simulink model "ADU_Integration_Y2016_simulation"  (R2016b)
settings: Solver=FixedStepDiscrete  StartTime=240  StopTime=300  FixedStep=0.01  RelTol=1e-3  EnableMultiTasking=on
PostLoadFcn:
  | , if any(exist('dsrtsu_mdlpostloadfcn', 'file') == [2, 3, 6]), try dsrtsu_mdlpostloadfcn('Execute', bdroot); catch fprintf('Error in PostLoadFcn (dsrtsu_mdlpostloadfcn) for model "%s":\n %s\n', bdroot, lasterr); end, end,
InitFcn:
  | load 'data/chi2_dat';
  | load 'data/innerLine_struct';
  | load 'data/middleLine_struct';
  | load 'data/outerLine_struct';
  | load 'data/innerLine';
  | load 'data/middleLine';
  | load 'data/outerLine';
  | load 'data/landmarks_patac_schimmel_ccw';
  | load 'data/patac_navi_array';
  | load 'data/sensor';
  | load 'data/map_struct';
  | addpath map_src
  | Integration_Parameter;
  | load 'TestData_001';
values from neighbouring files (symbols this model uses):
  TestData_001 =     [TestData_001.mat]
undefined symbols (not defined in the file or in its folder): a, chi2_dat, innerLine, landmarks_patac_schimmel_ccw, middleLine, outerLine, patac_navi_array, StartNum
libraries: simulink x36, rtican x1
(part 18 of 20)

== stateflow chart ADU_Integration_Y2016_simulation/LogData/RR_SRR_Data/Chart ==
  (default) -> (junction 13)
  (junction 13) -> (junction 14) [order 1] : [Trig != preTrig]
  (junction 13) -> (junction 15) [order 2]
  (junction 14) -> (junction 16) : {
      | DataOutput=DataInput;
      | Time_out=Time;
      | }
  (junction 16) -> (junction 15)
  (junction 15) -> (junction 17) : {
      | preTrig=Trig;
      | }
  data: Trig input; DataInput input size=[10 5]; DataOutput output double size=[10 5]; Time input; preTrig local double; Time_out output double

== matlab function ADU_Integration_Y2016_simulation/Path_Plan1/InterSectionPathPlanningModule/PathPrePointCal/PrePointCal ==
  data: V_tar input; Delta input; Arclength input; T_long input; T_lat input; Info_Me input; x_in input; y_in input; angle_in input; x_out input; y_out input; angle_out input; Time input; quadsinu2tbl data_store_memory; quadcosu2tbl data_store_memory; xposition output; yposition output; Ax output; Ay output; Vx output; Vy output; Theta output; PathPlanRes input; PathTrjFinishFlg output
function [xposition,yposition,Ax,Ay,Vx,Vy,Theta,PathTrjFinishFlg] = ElementaryPosCal( V_tar,Delta,Arclength,T_long,T_lat,Info_Me,x_in,y_in,angle_in,x_out,y_out,angle_out,Time,PathPlanRes)
%UNTITLED Summary of this function goes here
%   Detailed explanation goes here
persistent PrePointCalEn
if isempty(PrePointCalEn)
    PrePointCalEn = 0;
end
if PrePointCalEn <1e-1
    if PathPlanRes > 1e-1
        PrePointCalEn = 1;
    end
end
xposition = 0;yposition = 0;Ax = 0;Ay = 0;Vx = 0;Vy = 0;Theta = 0;PathTrjFinishFlg = 0;
    if PrePointCalEn > 1e-1
        V_me = Info_Me(3);
        Arc = 255;
        V_tarPos = 255;
        if Time > T_lat
        else
            if Time <= T_long
                if abs(V_tar - V_me) >1e-5
                    a_me = (V_tar - V_me)/T_long;
                else
                    a_me = 0;
                end
                Arc = V_me * Time + 0.5 * a_me * Time ^2;
                V_tarPos = V_me + Time * a_me;
            else
                Arc = (V_me + V_tar) /2 * T_long + (Time - T_long) * V_tar;            
                V_tarPos = V_tar;
            end
        end
        Beta = (angle_out - angle_in)/2;
        theta_rot = angle_in;
        x_outRot = (x_out - x_in)*cos(theta_rot) + (y_out - y_in)*sin(theta_rot);
        y_outRot = (y_out - y_in)*cos(theta_rot) - (x_out - x_in)*sin(theta_rot);    
        if Beta == 0
            SignBeta = 1;
        else
            SignBeta = sign(Beta);
        end
        if Arc < Arclength/2    
            ulimit = Arc * sqrt(abs(Delta)/2);
            Theta = Delta * (Arc)^2/2;
            xpositionTemp = sqrt(2/abs(Delta))*quadcosu2(ulimit);
            ypositionTemp = sqrt(2/abs(Delta))*quadsinu2(ulimit) * SignBeta;
            Kur = Arc * Delta;
        elseif Arc <= Arclength 
            ulimit = (Arclength - Arc) * sqrt(abs(Delta)/2); 
            %Theta = 2*Beta*SignBeta - Delta * (Arclength - Arc)^2/2; 
            xpositionMirrTemp = sqrt(2/abs(Delta))*quadcosu2(ulimit);
            ypositionMirrTemp = sqrt(2/abs(Delta))*quadsinu2(ulimit) * SignBeta;
            %mirror line Ax+By+C=0
            x_mirr = (x_outRot)/2;
            y_mirr = (y_outRot)/2;
            angle_mirr = pi/2 + atan((y_outRot)/(x_outRot));
            A = tan(angle_mirr);
            B = -1;
            C = y_mirr - A * x_mirr;      
            %two points are symmetrical to the Ax+By+C we just defined
            xpositionTemp = xpositionMirrTemp - 2*A*(A*xpositionMirrTemp+B*ypositionMirrTemp+C)/(A^2+B^2);
            ypositionTemp = ypositionMirrTemp - 2*B*(A*xpositionMirrTemp+B*ypositionMirrTemp+C)/(A^2+B^2);
            Theta = 2*abs(Beta)*SignBeta - Delta * (Arclength - Arc)^2/2; 
            Kur = Delta * Arc - Arclength/2 * Delta;
        else
            xpositionTemp = 0;ypositionTemp = 0;Kur = 0;Theta = 0;
            PrePointCalEn = 0;
            PathTrjFinishFlg = 1;
        end
        theta_rot = - angle_in;   
        xposition = xpositionTemp*cos(theta_rot) + ypositionTemp*sin(theta_rot);
        yposition = ypositionTemp*cos(theta_rot) - xpositionTemp*sin(theta_rot) ;  
        xposition = xposition + x_in;
        yposition = yposition + y_in;
        Theta = Theta + angle_in;    

        Vx = V_tarPos * cos(Theta);
        Vy = V_tarPos * sin(Theta);
        Arel = V_tarPos^2 * Kur;
        Ax = Arel * cos(Theta);
        Ay = Arel * sin(Theta);
    end
end

function quadcosu2val = quadcosu2( ulimit )
    %UNTITLED4 Summary of this function goes here
    %   Detailed explanation goes here
    % this function is used to calculate the integral of cos(x^2),which is used
    % to calculate x position
    global quadcosu2tbl
    index = fix(ulimit/0.0005) + 1;
    quadcosu2val = quadcosu2tbl(index);
end

function quadsinu2val = quadsinu2( ulimit )
%UNTITLED4 Summary of this function goes here
%   Detailed explanation goes here
% this function is used to calculate the integral of sin(x^2),which is used
% to calculate y position
    global quadsinu2tbl 
    index = fix(ulimit/0.0005) + 1;
    quadsinu2val = quadsinu2tbl(index);
end

== matlab function ADU_Integration_Y2016_simulation/Path_Plan1/InterSectionPathPlanningModule/PrePointCorConvert/CordConvter ==
  data: xpositionTar input; xpositionPre input; ypositionTar input; ypositionPre input; Ax input; Ay input; Vx input; Vy input; ThetaTar input; xpositionCur input; ypositionCur input; VsPathPlan_h_position output size=4; thetaCur input; VsPathPlan_h_Motion output size=4; ThetaLo output
function [VsPathPlan_h_position,VsPathPlan_h_Motion,ThetaLo] = ElementaryPosCal( xpositionTar,xpositionPre,ypositionTar,ypositionPre,Ax,Ay,Vx,Vy,ThetaTar,xpositionCur,ypositionCur,thetaCur )
%UNTITLED Summary of this function goes here
%   Detailed explanation goes here

    VsPathPlan_h_position = [0 0 0 0]';
    VsPathPlan_h_Motion = [0 0 0 0]';
    AfterRotX = [0 0 0 0];
    AfterRotY = [0 0 0 0];   
    
    BeforeRotX = [xpositionTar,xpositionPre,Ax,Vx];
    BeforeRotY = [ypositionTar,ypositionPre,Ay,Vy];   
    
    AfterRotX = (BeforeRotX - xpositionCur ) .* cos(thetaCur) + (BeforeRotY - ypositionCur ) .* sin(thetaCur);
    AfterRotY = (BeforeRotY - ypositionCur ) .* cos(thetaCur) - (BeforeRotX - xpositionCur ) .* sin(thetaCur);

    VsPathPlan_h_position(1) = AfterRotX(1);
    VsPathPlan_h_position(2) = AfterRotY(1);
    VsPathPlan_h_position(3) = AfterRotX(2);
    VsPathPlan_h_position(4) = AfterRotY(2);
    
    VsPathPlan_h_Motion(1) = AfterRotX(3);
    VsPathPlan_h_Motion(2) = AfterRotY(3);
    VsPathPlan_h_Motion(3) = AfterRotX(4);
    VsPathPlan_h_Motion(4) = AfterRotY(4);
    ThetaLo = ThetaTar - thetaCur;
    
end

== matlab function ADU_Integration_Y2016_simulation/Path_Plan1/LaneChangePathPlanningModule1/MATLAB Function ==
  data: CurOp input; TrigFlg output
function TrigFlg = OpTrigJudge(CurOp)
%#codegen
    %Operation 0 NA    %Operation 1 RT    %Operation 2 LT    %Operation 3 ST    %Operation 4 PK    %Operation 5 LC    %Operation 6 Transition
    persistent TrigEventEdge
    if isempty(TrigEventEdge)
        TrigEventEdge = 0;
    end
    TrigFlg = 0;
    if (abs(CurOp - 5)<1e-1)  
        TrigEdgeResCur = 1;
    else
        TrigEdgeResCur = 0;  
    end

    if ((abs(TrigEventEdge - TrigEdgeResCur) > 1e-1)) 
        if (TrigEdgeResCur > 1e-1)
            TrigFlg = 1;
        else
        end
        TrigEventEdge = TrigEdgeResCur;
    else
        TrigFlg = 0;
    end
end

== matlab function ADU_Integration_Y2016_simulation/Path_Plan1/LaneChangePathPlanningModule1/MATLAB Function1 ==
  data: RoadInfo input; x_in output; y_in output; angle_in output; x_out output; y_out output; angle_out output; W_in output; W_out output
function [x_in,y_in,angle_in,x_out,y_out,angle_out,W_in,W_out] = RoadInfoDistribute(RoadInfo)
%#codegen
%         RoadInfo(1,1) = Info_Me(1);RoadInfo(1,2) = Info_Me(2);RoadInfo(1,3) = Info_Me(6);RoadInfo(1,4) = EgoLaneInfo(2);
%         RoadInfo(2,:) = [EgoLaneInfo(3),EgoLaneInfo(4),EgoLaneInfo(1),EgoLaneInfo(2)]; 
    x_in = RoadInfo(1,1);y_in = RoadInfo(1,2);angle_in = RoadInfo(1,3);W_in = RoadInfo(1,4);
    x_out = RoadInfo(2,1);y_out = RoadInfo(2,2);angle_out = RoadInfo(2,3); W_out = RoadInfo(2,4);
end
